simulink model "volt_l_mfile"  (R2019a)
settings: Solver=VariableStepAuto  StartTime=0.0  StopTime=1  RelTol=1e-3
settings Model: Creator=USER  LastModifiedBy=USER
settings DataIOCC: ExternalInput=[0 0.016783]  InitialState=[]  LoadExternalInput=on  LoadInitialState=on
settings OptimizationCC: DefaultParameterBehavior=Inlined  BufferReuse=off
settings DebuggingCC: InitInArrayFormatMsg=none

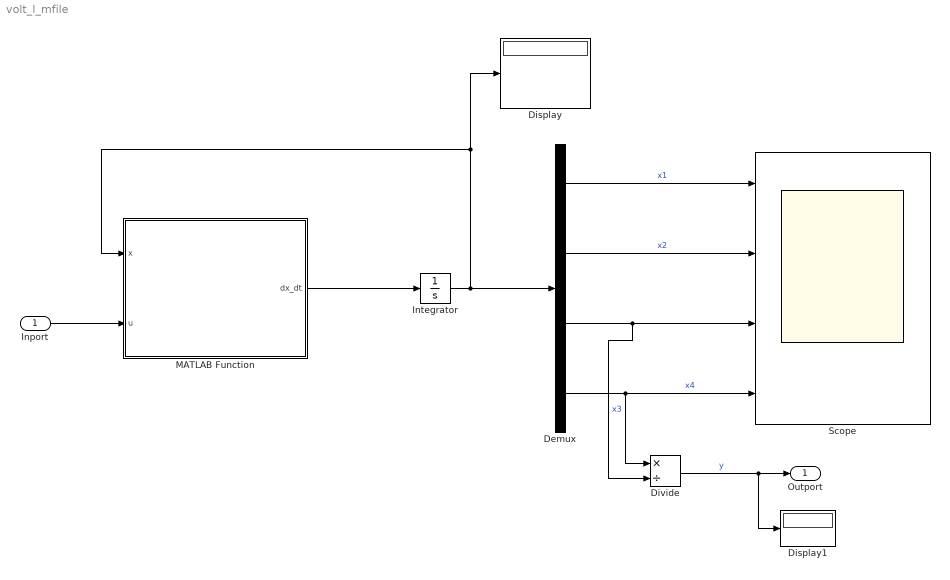
== system volt_l_mfile ==
  Inport : Inport
  Demux : Demux
  Display : Display
  Display1 : Display
  Divide : Product  Inputs=*/
  Integrator : Integrator  InitialCondition=[6,8,0,0]
  MATLAB Function : MATLAB Function  TreatAsAtomicUnit=on
  Scope : Scope  NumInputPorts=4
  Outport : Outport
  wires:
  MATLAB Function/1(dx_dt) -> Integrator/1
  Integrator/1 -> MATLAB Function/1(x), Display/1, Demux/1
  Inport/1 -> MATLAB Function/2(u)
  Demux/1 -> Scope/1  "x1"
  Demux/2 -> Scope/2  "x2"
  Demux/3 -> Divide/2, Scope/3  "x3"
  Demux/4 -> Divide/1, Scope/4  "x4"
  Divide/1 -> Outport/1, Display1/1  "y"

== matlab function volt_l_mfile/MATLAB Function ==
  data: x input; u input; dx_dt output
function dx_dt = volt(x,u)


%outputs
Cm = x(1);
Ci = x(2);
Do = x(3);
Di = x(4);

%inputs
Fi = u(1);

%initialize the differential equations
dx_dt = zeros(4,1);

%defining the differential equations

dx_dt(1) = 10*(6-Cm) - (2.4568*Cm*sqrt(Ci)); 
 
dx_dt(2) = 80*u - 10.1022*Ci;
 
dx_dt(3) = 0.0024121*Cm*sqrt(Ci) + 0.112191*Ci - 10*Do;
 
dx_dt(4) = 245.978*Cm*sqrt(Ci) - 10*Di;

y=u;
